simulink model "pfc_controller_codegen"  (R2025b)
settings: Solver=FixedStepDiscrete  StartTime=0.0  StopTime=0.5  FixedStep=Ts_ctrl  RelTol=1e-3
undefined symbols (not defined in the file): alpha, DiscIntNeverNeededParam, Ilimit, Izcd, K_Ton_max, Kff, Ki, Kp, Ncycle_min, Ton_max, Ton_min, Ton_startup_max, Ts_ctrl, Ts_v, Tstart, Vin_ff_max, Vin_ff_min, Vovp, Vref
libraries: simulink x8, eeGeneralControl x2
settings Model: Creator=nickj  LastModifiedBy=nickj
settings DataIOCC: SaveOutput=off  SaveTime=off  ReturnWorkspaceOutputsName=out_codegen  LoggingIntervals=[0, 0.5]
settings OptimizationCC: DefaultParameterBehavior=Inlined  EnhancedBackFolding=on  PassReuseOutputArgsAs=Individual arguments  ZeroExternalMemoryAtStartup=off  ZeroInternalMemoryAtStartup=off  MaxStackSize=512  OptimizeBlockOrder=speed  DifferentSizesBufferReuse=on  OptimizationCustomize=off  EfficientTunableParamExpr=on
settings DebuggingCC: ParameterTunabilityLossMsg=error
settings HardwareCC: ProdBitPerPointer=32.0  ProdBitPerSizeT=32.0  ProdBitPerPtrDiffT=32.0  ProdLargestAtomicInteger=Long  ProdLargestAtomicFloat=Double  ProdWordSize=32.0  ProdLongLongMode=on  ProdHWDeviceType=ARM Compatible->ARM Cortex-M
settings SFSimCC: MATLABDynamicMemAlloc=off
settings RTWCC: SystemTargetFile=ert.tlc  HardwareBoard=STM32G4xx Based  GenCodeOnly=on  TemplateMakefile=ert_default_tmf  GenerateReport=on  Toolchain=GNU Tools for ARM Embedded Processors  LaunchReport=on  GenerateTraceInfo=on  Description=Embedded Coder
settings CodeAppCC: ForceParamTrailComments=on  IgnoreCustomStorageClasses=off  OperatorAnnotations=on  SimulinkDataObjDesc=on  SFDataObjDesc=on  InsertBlockDesc=on
settings ERTTargetCC: ExtModeTransport=3.0  ExtModeStaticAlloc=on  ExtModeStaticAllocSize=2048.0  ExtModeMexFile=ext_xcp  ExtModeIntrfLevel=Level2 - Open  TargetLangStandard=C99 (ISO)  CodeReplacementLibrary=ARM Cortex-M

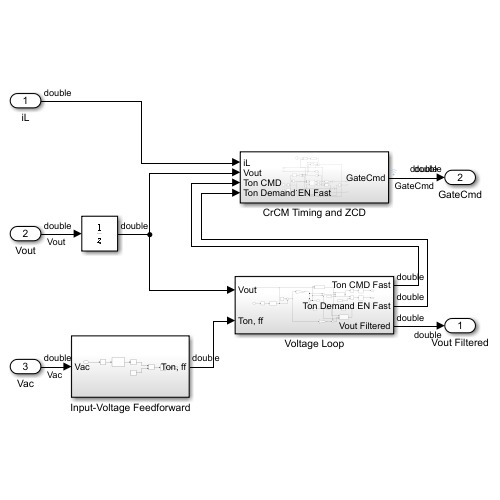
[thumbnail: Simulink's stored preview of the top-level diagram]
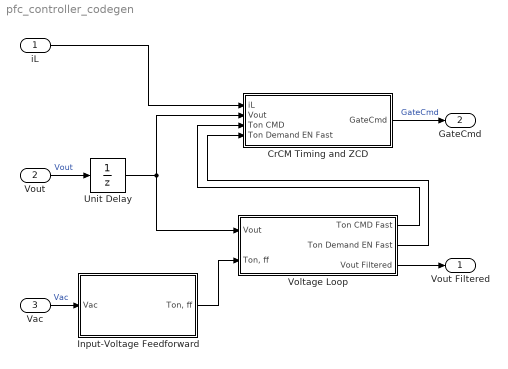
== system pfc_controller_codegen ==
  iL : Inport  OutDataTypeStr=double  PortDimensions=1  SampleTime=Ts_ctrl
  Vout : Inport  Port=2  OutDataTypeStr=double  PortDimensions=1  SampleTime=Ts_v
  Vac : Inport  Port=3  OutDataTypeStr=double  PortDimensions=1  SampleTime=Ts_v
  CrCM Timing and ZCD : Subsystem
  Input-Voltage Feedforward : Subsystem
  Unit Delay : UnitDelay  SampleTime=Ts_v  HasFrameUpgradeWarning=on
  Voltage Loop : Subsystem
  Vout Filtered : Outport  OutDataTypeStr=double  PortDimensions=1  SampleTime=[0.0001,0]
  GateCmd : Outport  Port=2  OutDataTypeStr=double  PortDimensions=1  SampleTime=[9.9999999999999995e-08,0]
  wires:
  iL/1 -> CrCM Timing and ZCD/1(iL)
  CrCM Timing and ZCD/1(GateCmd) -> GateCmd/1  "GateCmd"
  Voltage Loop/1(Ton CMD Fast) -> CrCM Timing and ZCD/3(Ton CMD)
  Vac/1 -> Input-Voltage Feedforward/1(Vac)  "Vac"
  Input-Voltage Feedforward/1("Ton, ff") -> Voltage Loop/2("Ton, ff")
  Voltage Loop/3(Vout Filtered) -> Vout Filtered/1
  Voltage Loop/2(Ton Demand EN Fast) -> CrCM Timing and ZCD/4(Ton Demand EN Fast)
  Vout/1 -> Unit Delay/1  "Vout"
  Unit Delay/1 -> CrCM Timing and ZCD/2(Vout), Voltage Loop/1(Vout)

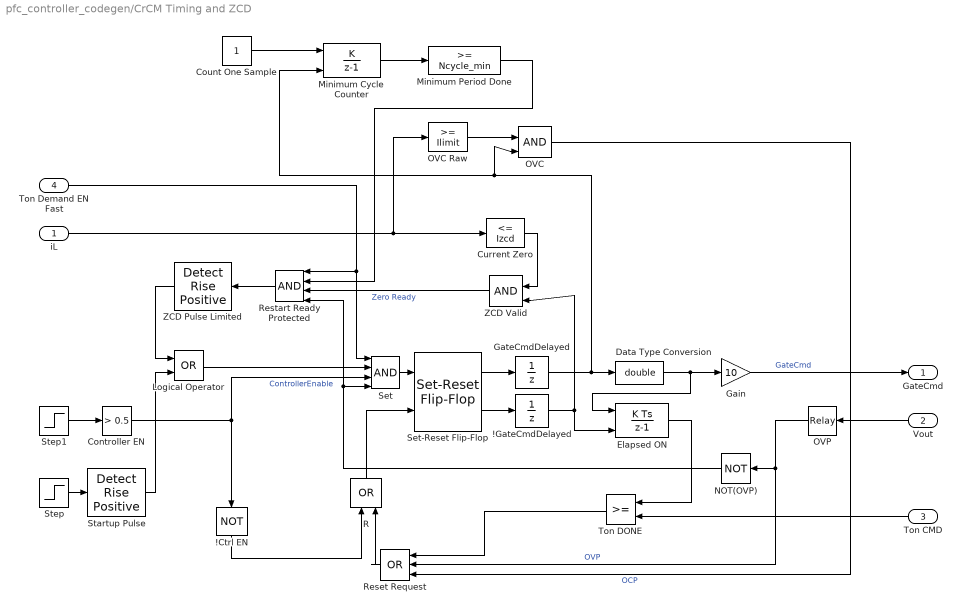
== system pfc_controller_codegen/CrCM Timing and ZCD ==
  iL : Inport
  Vout : Inport  Port=2
  Ton CMD : Inport  Port=3
  Ton Demand EN Fast : Inport  Port=4
  !Ctrl EN : Logic  Operator=NOT  IconShape=distinctive  AllPortsSameDT=off  OutDataTypeStr=boolean
  !GateCmdDelayed : UnitDelay  SampleTime=Ts_ctrl  HasFrameUpgradeWarning=on
  Controller EN : simulink/Logic and Bit Operations/Compare To Constant  relop=>  const=0.5  OutDataTypeStr=boolean
  Count One Sample : Constant  SampleTime=Ts_ctrl
  Current Zero : simulink/Logic and Bit Operations/Compare To Constant  relop=<=  const=Izcd  OutDataTypeStr=boolean
  Data Type Conversion : DataTypeConversion  OutDataTypeStr=double  SaturateOnIntegerOverflow=off  RndMeth=Floor
  Elapsed ON : DiscreteIntegrator  ExternalReset=level  SampleTime=Ts_ctrl  ICPrevOutput=DiscIntNeverNeededParam  ICPrevScaledInput=DiscIntNeverNeededParam
  Gain : Gain  Gain=10
  GateCmdDelayed : UnitDelay  SampleTime=Ts_ctrl  HasFrameUpgradeWarning=on
  Logical Operator : Logic  Operator=OR  AllPortsSameDT=off  OutDataTypeStr=boolean
  Minimum Cycle Counter : DiscreteIntegrator  IntegratorMethod=Accumulation: Forward Euler  ExternalReset=rising  SampleTime=Ts_ctrl  LimitOutput=on  UpperSaturationLimit=Ncycle_min  LowerSaturationLimit=0  ICPrevOutput=DiscIntNeverNeededParam  ICPrevScaledInput=DiscIntNeverNeededParam
  Minimum Period Done : simulink/Logic and Bit Operations/Compare To Constant  relop=>=  const=Ncycle_min  OutDataTypeStr=boolean
  NOT(OVP) : Logic  Operator=NOT  IconShape=distinctive  AllPortsSameDT=off  OutDataTypeStr=boolean
  OVC : Logic  IconShape=distinctive  AllPortsSameDT=off  OutDataTypeStr=boolean
  OVC Raw : simulink/Logic and Bit Operations/Compare To Constant  relop=>=  const=Ilimit  OutDataTypeStr=boolean
  OVP : Relay  OnSwitchValue=Vovp  OffSwitchValue=Vovp-10
  R : Logic  Operator=OR  IconShape=distinctive  AllPortsSameDT=off  OutDataTypeStr=boolean
  Reset Request : Logic  Operator=OR  Inputs=3  IconShape=distinctive  AllPortsSameDT=off  OutDataTypeStr=boolean
  Restart Ready Protected : Logic  Inputs=4  AllPortsSameDT=off  OutDataTypeStr=boolean
  Set : Logic  Inputs=4  AllPortsSameDT=off  OutDataTypeStr=boolean
  Set-Reset Flip-Flop : eeGeneralControl/Set-Reset Flip-Flop  LabelModeActiveChoice=Discrete  UndefState=Reset  Q0=0  Ts=Ts_ctrl
      settings: LibrarySourceBlock=ee_sl_lib/General Control/Set-Reset Flip-Flop
  Startup Pulse : simulink/Logic and Bit Operations/Detect Rise Positive  vinit=0  OutDataTypeStr=boolean
  Step : Step  Time=Tstart  SampleTime=Ts_ctrl
  Step1 : Step  Time=0.21  SampleTime=Ts_ctrl
  Ton DONE : RelationalOperator  OutDataTypeStr=boolean  RndMeth=Simplest  InputSameDT=off
  ZCD Pulse Limited : simulink/Logic and Bit Operations/Detect Rise Positive  vinit=0  OutDataTypeStr=boolean
  ZCD Valid : Logic  IconShape=distinctive  AllPortsSameDT=off  OutDataTypeStr=boolean
  GateCmd : Outport
  wires:
  Ton Demand EN Fast/1 -> Restart Ready Protected/1, Set/1
  Restart Ready Protected/1 -> ZCD Pulse Limited/1
  GateCmdDelayed/1 -> Data Type Conversion/1, OVC/2, Minimum Cycle Counter/2
  Count One Sample/1 -> Minimum Cycle Counter/1
  Minimum Cycle Counter/1 -> Minimum Period Done/1
  Minimum Period Done/1 -> Restart Ready Protected/2
  !Ctrl EN/1 -> R/1
  Reset Request/1 -> R/2
  R/1 -> Set-Reset Flip-Flop/2
  Controller EN/1 -> Set/3, !Ctrl EN/1  "ControllerEnable"
  Step1/1 -> Controller EN/1
  Set/1 -> Set-Reset Flip-Flop/1
  Ton CMD/1 -> Ton DONE/2
  Ton DONE/1 -> Reset Request/1
  Elapsed ON/1 -> Ton DONE/1
  !GateCmdDelayed/1 -> Elapsed ON/2, ZCD Valid/2
  Set-Reset Flip-Flop/2 -> !GateCmdDelayed/1
  Gain/1 -> GateCmd/1  "GateCmd"
  Vout/1 -> OVP/1
  Data Type Conversion/1 -> Gain/1, Elapsed ON/1
  Logical Operator/1 -> Set/2
  NOT(OVP)/1 -> Restart Ready Protected/4, Set/4
  ZCD Pulse Limited/1 -> Logical Operator/1
  OVC/1 -> Reset Request/3  "OCP"
  OVC Raw/1 -> OVC/1
  ZCD Valid/1 -> Restart Ready Protected/3  "Zero Ready"
  Current Zero/1 -> ZCD Valid/1
  OVP/1 -> NOT(OVP)/1, Reset Request/2  "OVP"
  Set-Reset Flip-Flop/1 -> GateCmdDelayed/1
  iL/1 -> OVC Raw/1, Current Zero/1
  Step/1 -> Startup Pulse/1
  Startup Pulse/1 -> Logical Operator/2

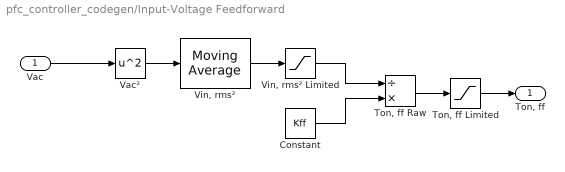
== system pfc_controller_codegen/Input-Voltage Feedforward ==
  Vac : Inport  SampleTime=Ts_v
  Constant : Constant  Value=Kff
  "Ton, ff Limited" : Saturate  UpperLimit=Ton_max  LowerLimit=Ton_min
  "Ton, ff Raw" : Product  Inputs=/*
  Vac² : Math  Operator=square
  "Vin, rms²" : eeGeneralControl/Moving Average  VariantControl=Variant1  LabelModeActiveChoice=Discrete  f=Favg  x0=Vin_ff_max^2  BufferSize=8192  Ts=Ts_v
      settings: LibrarySourceBlock=ee_sl_lib/General Control/Moving Average
  "Vin, rms² Limited" : Saturate  UpperLimit=Vin_ff_max^2  LowerLimit=Vin_ff_min^2
  "Ton, ff" : Outport
  wires:
  "Vin, rms² Limited"/1 -> "Ton, ff Raw"/1
  "Vin, rms²"/1 -> "Vin, rms² Limited"/1
  Vac²/1 -> "Vin, rms²"/1
  Vac/1 -> Vac²/1
  Constant/1 -> "Ton, ff Raw"/2
  "Ton, ff Raw"/1 -> "Ton, ff Limited"/1
  "Ton, ff Limited"/1 -> "Ton, ff"/1

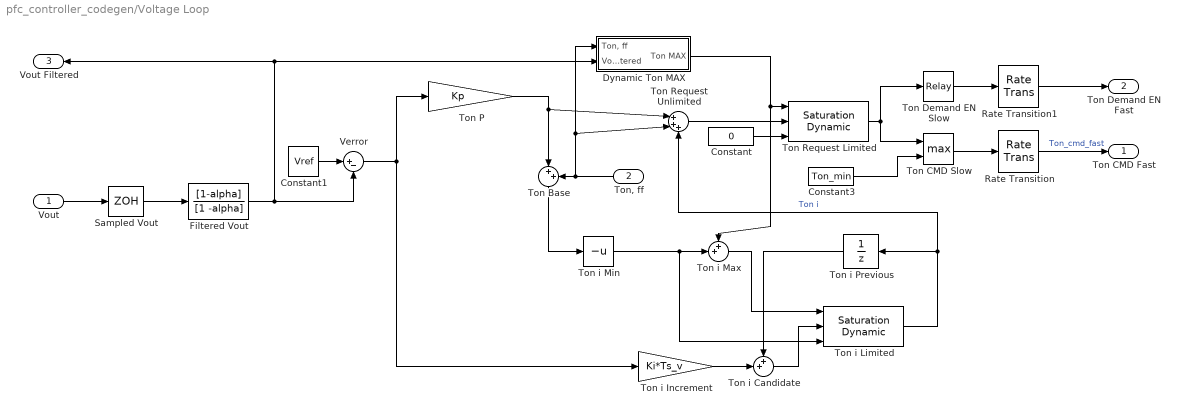
== system pfc_controller_codegen/Voltage Loop ==
  Vout : Inport  SampleTime=Ts_v
  "Ton, ff" : Inport  Port=2
  Constant : Constant  Value=0
  Constant1 : Constant  Value=Vref
  Constant3 : Constant  Value=Ton_min
  Dynamic Ton MAX : Subsystem
  Filtered Vout : DiscreteFilter  Numerator=[1-alpha]  Denominator=[1 -alpha]
  Rate Transition : RateTransition  OutPortSampleTime=Ts_ctrl
  Rate Transition1 : RateTransition  OutPortSampleTime=Ts_ctrl
  Sampled Vout : ZeroOrderHold  SampleTime=Ts_v
  Ton Base : Sum  Inputs=|++
  Ton CMD Slow : MinMax  Function=max  Inputs=2
  Ton Demand EN Slow : Relay  OnSwitchValue=0.25e-6  OffSwitchValue=0.15e-6
  Ton P : Gain  Gain=Kp
  Ton Request Limited : simulink/Discontinuities/Saturation Dynamic  OutMin=[]  OutMax=[]  OutDataTypeStr=Inherit: Same as second input  OutDataType=fixdt(1, 16)  OutScaling=2^-10  DoSatur=off
  Ton Request Unlimited : Sum  Inputs=|+++
  Ton i Candidate : Sum  Inputs=++|
  Ton i Increment : Gain  Gain=Ki*Ts_v
  Ton i Limited : simulink/Discontinuities/Saturation Dynamic  OutMin=[]  OutMax=[]  OutDataTypeStr=Inherit: Same as second input  OutDataType=fixdt(1, 16)  OutScaling=2^-10  DoSatur=off
  Ton i Max : Sum  Inputs=++|
  Ton i Min : UnaryMinus
  Ton i Previous : UnitDelay  SampleTime=Ts_v  HasFrameUpgradeWarning=on
  Verror : Sum  Inputs=|+-
  Ton CMD Fast : Outport
  Ton Demand EN Fast : Outport  Port=2
  Vout Filtered : Outport  Port=3
  wires:
  Rate Transition1/1 -> Ton Demand EN Fast/1
  Ton Demand EN Slow/1 -> Rate Transition1/1
  Ton CMD Slow/1 -> Rate Transition/1
  Constant3/1 -> Ton CMD Slow/2
  Ton Request Limited/1 -> Ton CMD Slow/1, Ton Demand EN Slow/1
  Ton i Increment/1 -> Ton i Candidate/2
  Ton i Previous/1 -> Ton i Candidate/1
  Ton i Limited/1 -> Ton Request Unlimited/3, Ton i Previous/1  "Ton i"
  Ton i Candidate/1 -> Ton i Limited/2
  Ton i Min/1 -> Ton i Limited/3, Ton i Max/2
  Ton i Max/1 -> Ton i Limited/1
  Ton Base/1 -> Ton i Min/1
  Dynamic Ton MAX/1(Ton MAX) -> Ton Request Limited/1, Ton i Max/1
  Constant/1 -> Ton Request Limited/3
  "Ton, ff"/1 -> Ton Request Unlimited/2, Dynamic Ton MAX/1("Ton, ff"), Ton Base/2
  Vout/1 -> Sampled Vout/1
  Ton P/1 -> Ton Request Unlimited/1, Ton Base/1
  Constant1/1 -> Verror/1
  Sampled Vout/1 -> Filtered Vout/1
  Rate Transition/1 -> Ton CMD Fast/1  "Ton_cmd_fast"
  Ton Request Unlimited/1 -> Ton Request Limited/2
  Verror/1 -> Ton i Increment/1, Ton P/1
  Filtered Vout/1 -> Vout Filtered/1, Dynamic Ton MAX/2(Vout Filtered), Verror/2

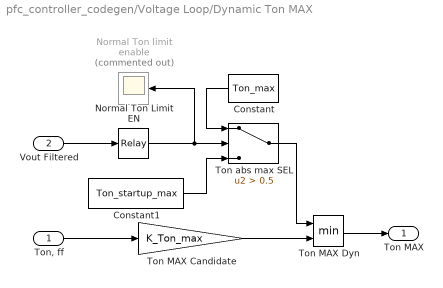
== system pfc_controller_codegen/Voltage Loop/Dynamic Ton MAX ==
  "Ton, ff" : Inport
  Vout Filtered : Inport  Port=2
  Constant : Constant  Value=Ton_max
  Constant1 : Constant  Value=Ton_startup_max
  Normal Ton Limit EN : Relay  OnSwitchValue=390  OffSwitchValue=370
  Normal Ton limit enable : Scope  Commented=on
      settings: ActiveDisplayYMinimum=-1  ActiveDisplayYMaximum=1  DataLoggingVariableName=ScopeData8
  Ton MAX Candidate : Gain  Gain=K_Ton_max
  Ton MAX Dyn : MinMax  Inputs=2
  Ton abs max SEL : Switch  Criteria=u2 > Threshold  Threshold=0.5  SaturateOnIntegerOverflow=off  InputSameDT=off
  Ton MAX : Outport
  wires:
  Vout Filtered/1 -> Normal Ton Limit EN/1
  Constant/1 -> Ton abs max SEL/1
  Constant1/1 -> Ton abs max SEL/3
  Ton abs max SEL/1 -> Ton MAX Dyn/1
  Normal Ton Limit EN/1 -> Ton abs max SEL/2, Normal Ton limit enable/1
  "Ton, ff"/1 -> Ton MAX Candidate/1
  Ton MAX Candidate/1 -> Ton MAX Dyn/2
  Ton MAX Dyn/1 -> Ton MAX/1
